simulink model "SD2231_Lab1_2022"  (R2020b)
settings: Solver=VariableStepAuto  StartTime=0.0  StopTime=inf  RelTol=1e-3
values from neighbouring files (symbols this model uses):
  delay = 250    [initial.m]
  K_awup = Ki_br_r/Kp_br_r    (= 10.4166666667)    [initial.m]
  K_brake = K_brake(3)    [initial.m]
  K_em = K_em(3)    [initial.m]
  Kd_br_f = 0*0.6*T_new_rl_b    (= 0)    [initial.m]
  Kd_br_r = 0.6*T_new_rl_b    (= 0.1722)    [initial.m]
  Kd_tr = 0.6*T_new    (= 0.0093)    [initial.m]
  Ki_br_f = 0.5*0.6*T_new_rl_b/L_new_rl_b^2    (= 37.3697916667)    [initial.m]
  Ki_br_r = 0.6*T_new_rl_b/L_new_rl_b^2    (= 74.7395833333)    [initial.m]
  Ki_tr = 0.6*T_new/L_new^2    (= 4.12188365651)    [initial.m]
  Kp_br_f = 1.2*T_new_rl_b/L_new_rl_b    (= 7.175)    [initial.m]
  Kp_br_r = 1.2*T_new_rl_b/L_new_rl_b    (= 7.175)    [initial.m]
  Kp_tr = 2.2*1.2*T_new/L_new    (= 0.861473684211)    [initial.m]
  N = 100    [initial.m]
  ref_br_f = 0.15    [initial.m]
  ref_br_r = 0.17-0.1    (= 0.07)    [initial.m]
  ref_tr = 0.06    [initial.m]
  step_time = 2    [initial.m]
  threshold_br_f = ref_br_f-0.05    (= 0.1)    [initial.m]
  threshold_br_r = ref_br_r-0.05    (= 0.02)    [initial.m]
  threshold_tc = ref_tr-0.02    (= 0.04)    [initial.m]
  vx_threshold = 1    [initial.m]
undefined symbols (not defined in the file or in its folder): DiscIntNeverNeededParam, Veh
libraries: CarMaker4SL x38, simulink x2, autolibmappedmotor x2
(part 4 of 4)

== system SD2231_Lab1_2022/CarMaker/IPG Vehicle/PowerTrain/User RearDriven PowerTrain1/RR Motor ==
  Gas : Inport
  "Motor speed " : Inport  Port=2
  Mapped Motor : autolibmappedmotor/Mapped Motor  port_config=Speed  param_by=Tabulated torque-speed envelope  w_t=[ 0 500 5000 10000 16000]  T_t=[440 440 350 300 280]  torque_max=.1  power_max=30  Tc=0.02  param_loss=Single efficiency measurement  eff=100  w_eff=375  T_eff=440  Piron=0  Pbase=0  w_eff_bp=[-8000 -4000 0 4000 8000]  T_eff_bp=[0 0.03 0.06 0.09]  Temp_eff_bp=[233.15 293.15 373.15]  losses_table=[1.49 1.67 2.21 3.10; 0.42 0.69 1.14 2.03; 0.06 0.24 0.78 1.68; 0.42 0.69 1.14 2.03; 1.49 1.67 2.21 3.10]  losses_table_3d=cat(3,1.05*[1.49 1.67 2.21 3.10; 0.42 0.69 1.14 2.03; 0.06 0.24 0.78 1.68; 0.42 0.69 1.14 2.03; 1.49 1.67 2.21 3.10],[1.49 1.67 2.21 3.10; 0.42 0.69 1.14 2.03; 0.06 0.24 0.78 1.68; 0.42 0.69 1.14 2.03; 1.49 1.67 2.21 3.10],1.03*[1.49 1.67 2.21 3.10; 0.42 0.69 1.14 2.03; 0.06 0.24 0.78 1.68; 0.42 0.69 1.14 2.03; 1.49 1.67 2.21 3.10])  efficiency_table=[95 95 95 95; 95 95 95 95; 95 95 95 95; 95 95 95 95; 95 95 95 95]  efficiency_table_3d=cat(3,90*ones(5,4),95*ones(5,4),92*ones(5,4))  J=0.002  b=1e-5  omega_o=0  T_t_extended=[280 300 350 440 440 440 350 300 280]  w_t_extended=[-16000 -10000 -5000 -500 0 500 5000 10000 16000]  KLossIron=0  KLossCopper=0  x_w_eff_vec=[-8000 -4000 0 4000 8000]  x_T_eff_vec=[-0.09 -0.06 -0.03 0 0.03 0.06 0.09]  x_tmp_eff_vec=[233.15 293.15 373.15]  x_losses_mat=[3.1 2.21 1.67 1.49 1.67 2.21 3.1;2.03 1.14 0.69 0.42 0.69 1.14 2.03;1.68 0.78 0.24 0.06 0.24 0.78 1.68;2.03 1.14 0.69 0.42 0.69 1.14 2.03;3.1 2.21 1.67 1.49 1.67 2.21 3.1]  x_losses_mat_3d=cat(3,[3.255 2.3205 1.7535 1.5645 1.7535 2.3205 3.255;2.1315 1.197 0.7245 0.441 0.7245 1.197 2.1315;1.764 0.819 0.252 0.063 0.252 0.819 1.764;2.1315 1.197 0.7245 0.441 0.7245 1.197 2.1315;3.255 2.3205 1.7535 1.5645 1.7535 2.3205 3.255],[3.1 2.21 1.67 1.49 1.67 2.21 3.1;2.03 1.14 0.69 0.42 0.69 1.14 2.03;1.68 0.78 0.24 0.06 0.24 0.78 1.68;2.03 1.14 0.69 0.42 0.69 1.14 2.03;3.1 2.21 1.67 1.49 1.67 2.21 3.1],[3.193 2.2763 1.7201 1.5347 1.7201 2.2763 3.193;2.0909 1.1742 0.7107 0.4326 0.7107 1.1742 2.0909;1.7304 0.8034 0.2472 0.0618 0.2472 0.8034 1.7304;2.0909 1.1742 0.7107 0.4326 0.7107 1.1742 2.0909;3.193 2.2763 1.7201 1.5347 1.7201 2.2763 3.193])  CalLossMapData={}  CalLossWithTempMapData={}  aMode=2  RefBlkName='autolibmappedmotor/Mapped Motor'
      settings: SourceProductBaseCode=PW
  "Max Torque from motor " : Constant  Value=K_em
  Product : Product  RndMeth=Zero
  Read CM Dict : CarMaker4SL/Read CM Dict  xname=PT.BattHV.Volt_oc  xsync=off  xstime=Continuous
  Scope : Scope
  Terminator : Terminator
  Terminator1 : Terminator
  Motor Trq : Outport  VectorParamsAs1DForOutWhenUnconnected=off
  wires:
  Mapped Motor/3 -> Motor Trq/1
  Read CM Dict/1 -> Mapped Motor/1
  Gas/1 -> Product/1
  Product/1 -> Mapped Motor/3
  "Max Torque from motor "/1 -> Product/2
  Mapped Motor/1 -> Terminator/1
  Mapped Motor/2 -> Terminator1/1
  "Motor speed "/1 -> Scope/1, Mapped Motor/2

== system SD2231_Lab1_2022/CarMaker/IPG Vehicle/PowerTrain/User RearDriven PowerTrain1/Subsystem ==
  LR motor Torque : Inport
  RR motor Torque : Inport  Port=2
  Gear ratio : Gain  Gain=9.73
  Gear ratio1 : Gain  Gain=9.73
  "LRTrq " : Outport  VectorParamsAs1DForOutWhenUnconnected=off
  RRTrq : Outport  Port=2  VectorParamsAs1DForOutWhenUnconnected=off
  wires:
  LR motor Torque/1 -> Gear ratio1/1
  RR motor Torque/1 -> Gear ratio/1
  Gear ratio/1 -> RRTrq/1
  Gear ratio1/1 -> "LRTrq "/1

== system SD2231_Lab1_2022/CarMaker/IPG Vehicle/PowerTrain/User RearDriven PowerTrain1/WheelInertia ==
  In1 : Inport
  Divide : Product  Inputs=*/
  Read CM Parameter : CarMaker4SL/Read CM Parameter  xfile=Vehicle  xkey=Wheel.fl.I  xnout=3  xdefaults=[]  xmuxed=off  xstime=Continuous
      settings: SourceProductName=CarMaker4SL
  Switch : Switch  Criteria=u2 ~= 0  ZeroCross=off
  Terminator : Terminator
  Terminator1 : Terminator
  Zero : Constant
  Out1 : Outport  VectorParamsAs1DForOutWhenUnconnected=off
  wires:
  Read CM Parameter/2 -> Switch/1, Switch/2
  Switch/1 -> Divide/2
  Zero/1 -> Switch/3
  In1/1 -> Divide/1
  Read CM Parameter/3 -> Terminator1/1
  Read CM Parameter/1 -> Terminator/1
  Divide/1 -> Out1/1

== system SD2231_Lab1_2022/CarMaker/IPG Vehicle/PowerTrain/User RearDriven PowerTrain1/WheelInertia1 ==
  In1 : Inport
  Divide : Product  Inputs=*/
  Read CM Parameter : CarMaker4SL/Read CM Parameter  xfile=Vehicle  xkey=Wheel.fr.I  xnout=3  xdefaults=[]  xmuxed=off  xstime=Continuous
      settings: SourceProductName=CarMaker4SL
  Switch : Switch  Criteria=u2 ~= 0  ZeroCross=off
  Terminator : Terminator
  Terminator1 : Terminator
  Zero : Constant
  Out1 : Outport  VectorParamsAs1DForOutWhenUnconnected=off
  wires:
  Divide/1 -> Out1/1
  Read CM Parameter/1 -> Terminator/1
  Read CM Parameter/3 -> Terminator1/1
  In1/1 -> Divide/1
  Read CM Parameter/2 -> Switch/2, Switch/1
  Zero/1 -> Switch/3
  Switch/1 -> Divide/2

== system SD2231_Lab1_2022/CarMaker/IPG Vehicle/PowerTrain/User RearDriven PowerTrain1/WheelInertia2 ==
  In1 : Inport
  Divide : Product  Inputs=*/
  Read CM Parameter : CarMaker4SL/Read CM Parameter  xfile=Vehicle  xkey=Wheel.rl.I  xnout=3  xdefaults=[]  xmuxed=off  xstime=Continuous
      settings: SourceProductName=CarMaker4SL
  Switch : Switch  Criteria=u2 ~= 0  ZeroCross=off
  Terminator : Terminator
  Terminator1 : Terminator
  Zero : Constant
  Out1 : Outport  VectorParamsAs1DForOutWhenUnconnected=off
  wires:
  Switch/1 -> Divide/2
  Zero/1 -> Switch/3
  Read CM Parameter/2 -> Switch/1, Switch/2
  In1/1 -> Divide/1
  Read CM Parameter/3 -> Terminator1/1
  Read CM Parameter/1 -> Terminator/1
  Divide/1 -> Out1/1

== system SD2231_Lab1_2022/CarMaker/IPG Vehicle/PowerTrain/User RearDriven PowerTrain1/WheelInertia3 ==
  In1 : Inport
  Divide : Product  Inputs=*/
  Read CM Parameter : CarMaker4SL/Read CM Parameter  xfile=Vehicle  xkey=Wheel.rr.I  xnout=3  xdefaults=[]  xmuxed=off  xstime=Continuous
      settings: SourceProductName=CarMaker4SL
  Switch : Switch  Criteria=u2 ~= 0  ZeroCross=off
  Terminator : Terminator
  Terminator1 : Terminator
  Zero : Constant
  Out1 : Outport  VectorParamsAs1DForOutWhenUnconnected=off
  wires:
  Divide/1 -> Out1/1
  Read CM Parameter/1 -> Terminator/1
  Read CM Parameter/3 -> Terminator1/1
  In1/1 -> Divide/1
  Read CM Parameter/2 -> Switch/2, Switch/1
  Zero/1 -> Switch/3
  Switch/1 -> Divide/2

== system SD2231_Lab1_2022/CarMaker/Your ABS Controller/Activation Logic Br FL/Subsystem/PID1 ==
  err : Inport
  Brake Pedal : Inport  Port=2
  slip : Inport  Port=3
  Add : Sum
  Add1 : Sum  Inputs=-+
  Add2 : Sum
  Brake Pedal1 : InportShadow  Port=2
  Constant : Constant  Value=0
  Constant1 : Constant  Value=0
  Constant2 : Constant  Value=threshold_br_f
  Integrator : Integrator
  Integrator1 : Integrator
  Kd : Gain  Gain=Kd_br_f
  Ki : Gain  Gain=Ki_br_f
  Ki1 : Gain  Gain=K_awup
  MATLAB Function : MATLAB Function  TreatAsAtomicUnit=on
  Manual Switch : ManualSwitch  CurrentSetting=0
  N : Gain  Gain=N
  PID FL : Scope  NumInputPorts=4
  Saturation : Saturate  UpperLimit=1  LowerLimit=0
  Scope1 : Scope  NumInputPorts=2
  Sum : Sum  Inputs=|+-
  Sum1 : Sum  Inputs=+|+|+
  Switch : Switch  Criteria=u2 > Threshold  Threshold=0.5
  kp : Gain  Gain=Kp_br_f
  AdjBrk : Outport
  wires:
  kp/1 -> PID FL/1, Sum1/1  "KP"
  Integrator1/1 -> Sum/2
  N/1 -> Integrator1/1, Sum1/3, PID FL/3  "KD"
  Sum/1 -> N/1
  Kd/1 -> Sum/1
  Integrator/1 -> PID FL/2, Sum1/2  "KI"
  err/1 -> Switch/1, PID FL/4, kp/1, Kd/1  "err"
  Sum1/1 -> Add/1, AdjBrk/1
  Brake Pedal/1 -> Add/2
  Add/1 -> Add1/1, Saturation/1
  Saturation/1 -> Add1/2
  Add1/1 -> Ki1/1
  Ki/1 -> Scope1/1, Add2/1
  Add2/1 -> Integrator/1
  Manual Switch/1 -> Add2/2
  Constant/1 -> Manual Switch/1
  Ki1/1 -> Scope1/2, Manual Switch/2
  Switch/1 -> Ki/1  "err_slip"
  Constant1/1 -> Switch/3
  MATLAB Function/1(res) -> Switch/2
  slip/1 -> MATLAB Function/2(slip)
  Brake Pedal1/1 -> MATLAB Function/3(Brk)
  Constant2/1 -> MATLAB Function/1(threshold_br_r)

== system SD2231_Lab1_2022/CarMaker/Your ABS Controller/Activation Logic Br FR/Subsystem/PID ==
  err : Inport
  res : Inport  Port=2
  Integrator : Integrator  ExternalReset=rising
  Integrator1 : Integrator
  Kd : Gain  Gain=Kd_br_f
  Ki : Gain  Gain=Ki_br_f
  N : Gain  Gain=N
  Sum : Sum  Inputs=|+-
  Sum1 : Sum  Inputs=+|+|+
  kp : Gain  Gain=Kp_br_f
  Out1 : Outport
  wires:
  err/1 -> Kd/1, Ki/1, kp/1
  Ki/1 -> Integrator/1
  Kd/1 -> Sum/1
  Sum/1 -> N/1
  N/1 -> Sum1/3, Integrator1/1
  Integrator1/1 -> Sum/2
  Integrator/1 -> Sum1/2
  kp/1 -> Sum1/1
  Sum1/1 -> Out1/1
  res/1 -> Integrator/2

== system SD2231_Lab1_2022/CarMaker/Your ABS Controller/Activation Logic Br FR/Subsystem1/PID1 ==
  err : Inport
  Brake Pedal : Inport  Port=2
  slip : Inport  Port=3
  Add : Sum
  Add1 : Sum  Inputs=-+
  Add2 : Sum
  Brake Pedal1 : InportShadow  Port=2
  Constant : Constant  Value=0
  Constant1 : Constant  Value=0
  Constant2 : Constant  Value=threshold_br_f
  Integrator : Integrator
  Integrator1 : Integrator
  Kd : Gain  Gain=Kd_br_f
  Ki : Gain  Gain=Ki_br_f
  Ki1 : Gain  Gain=K_awup
  MATLAB Function1 : MATLAB Function  TreatAsAtomicUnit=on
  Manual Switch : ManualSwitch  CurrentSetting=0
  N : Gain  Gain=N
  Saturation : Saturate  UpperLimit=1  LowerLimit=0
  Scope : Scope  NumInputPorts=4
  Scope1 : Scope  NumInputPorts=2
  Sum : Sum  Inputs=|+-
  Sum1 : Sum  Inputs=+|+|+
  Switch : Switch  Criteria=u2 > Threshold  Threshold=0.5
  kp : Gain  Gain=Kp_br_f
  AdjBrk : Outport
  wires:
  kp/1 -> Scope/1, Sum1/1  "KP"
  Integrator1/1 -> Sum/2
  N/1 -> Integrator1/1, Sum1/3, Scope/3  "KD"
  Sum/1 -> N/1
  Kd/1 -> Sum/1
  Integrator/1 -> Scope/2, Sum1/2  "KI"
  Sum1/1 -> Add/1, AdjBrk/1
  Brake Pedal/1 -> Add/2
  Add/1 -> Add1/1, Saturation/1
  Saturation/1 -> Add1/2
  Add1/1 -> Ki1/1
  Ki/1 -> Scope1/1, Add2/1
  Add2/1 -> Integrator/1
  Manual Switch/1 -> Add2/2
  Constant/1 -> Manual Switch/1
  Ki1/1 -> Scope1/2, Manual Switch/2
  Constant1/1 -> Switch/3
  err/1 -> Switch/1, Scope/4, kp/1, Kd/1  "err_slip"
  Switch/1 -> Ki/1  "err_slip"
  slip/1 -> MATLAB Function1/2(slip)
  Brake Pedal1/1 -> MATLAB Function1/3(Brk)
  MATLAB Function1/1(res) -> Switch/2
  Constant2/1 -> MATLAB Function1/1(threshold_br_r)

== system SD2231_Lab1_2022/CarMaker/Your ABS Controller/Activation Logic Br RL/Subsystem/PID1 ==
  err : Inport
  slip : Inport  Port=2
  Brake Pedal : Inport  Port=3
  Add : Sum
  Add1 : Sum  Inputs=-+
  Add2 : Sum
  Brake Pedal1 : InportShadow  Port=3
  Constant : Constant  Value=0
  Constant1 : Constant  Value=0
  Constant2 : Constant  Value=threshold_br_r
  Integrator : Integrator
  Integrator1 : Integrator
  Kd : Gain  Gain=Kd_br_r
  Ki : Gain  Gain=Ki_br_r
  Ki1 : Gain  Gain=K_awup
  MATLAB Function : MATLAB Function  TreatAsAtomicUnit=on
  Manual Switch : ManualSwitch  CurrentSetting=0
  N : Gain  Gain=N
  PID FL : Scope  NumInputPorts=4
  Saturation : Saturate  UpperLimit=1  LowerLimit=0
  Scope1 : Scope  NumInputPorts=2
  Sum : Sum  Inputs=|+-
  Sum1 : Sum  Inputs=+|+|+
  Switch : Switch  Criteria=u2 > Threshold  Threshold=0.5
  kp : Gain  Gain=Kp_br_r
  AdjBrk : Outport
  wires:
  kp/1 -> PID FL/1, Sum1/1  "KP"
  Integrator1/1 -> Sum/2
  N/1 -> Integrator1/1, Sum1/3, PID FL/3  "KD"
  Sum/1 -> N/1
  Kd/1 -> Sum/1
  Integrator/1 -> PID FL/2, Sum1/2  "KI"
  err/1 -> Switch/1, PID FL/4, kp/1, Kd/1  "err"
  Sum1/1 -> Add/1, AdjBrk/1
  Brake Pedal/1 -> Add/2
  Add/1 -> Add1/1, Saturation/1
  Saturation/1 -> Add1/2
  Add1/1 -> Ki1/1
  Ki/1 -> Scope1/1, Add2/1
  Add2/1 -> Integrator/1
  Manual Switch/1 -> Add2/2
  Constant/1 -> Manual Switch/1
  Ki1/1 -> Scope1/2, Manual Switch/2
  Switch/1 -> Ki/1  "err_slip"
  Constant1/1 -> Switch/3
  Brake Pedal1/1 -> MATLAB Function/3(Brk)
  MATLAB Function/1(res) -> Switch/2
  slip/1 -> MATLAB Function/2(slip)
  Constant2/1 -> MATLAB Function/1(threshold_br_r)  "threshold_br_r"

== system SD2231_Lab1_2022/CarMaker/Your ABS Controller/Activation Logic Br RL old/Subsystem/PID ==
  err : Inport
  res : Inport  Port=2
  Integrator : Integrator  ExternalReset=rising
  Integrator1 : Integrator
  Kd : Gain  Gain=Kd_br_r
  Ki : Gain  Gain=Ki_br_r
  N : Gain  Gain=N
  Sum : Sum  Inputs=|+-
  Sum1 : Sum  Inputs=+|+|+
  kp : Gain  Gain=Kp_br_r
  Out1 : Outport
  wires:
  err/1 -> Kd/1, Ki/1, kp/1
  Ki/1 -> Integrator/1
  Kd/1 -> Sum/1
  Sum/1 -> N/1
  N/1 -> Sum1/3, Integrator1/1
  Integrator1/1 -> Sum/2
  Integrator/1 -> Sum1/2
  kp/1 -> Sum1/1
  Sum1/1 -> Out1/1
  res/1 -> Integrator/2

== system SD2231_Lab1_2022/CarMaker/Your ABS Controller/Activation Logic Br RL old 2/Controller/PID ==
  err : Inport
  Brake Pedal : Inport  Port=2
  Add : Sum
  Add1 : Sum  Inputs=-+
  Add2 : Sum
  Brake Pedal1 : InportShadow  Port=2
  Constant : Constant  Value=0
  Constant1 : Constant  Value=0
  Integrator : Integrator
  Integrator1 : Integrator
  Kd : Gain  Gain=Kd_br_r
  Ki : Gain  Gain=Ki_br_r
  Ki1 : Gain  Gain=K_awup
  MATLAB Function : MATLAB Function  TreatAsAtomicUnit=on
  Manual Switch : ManualSwitch
  N : Gain  Gain=N
  PID RL : Scope  NumInputPorts=4
  Saturation : Saturate  UpperLimit=1  LowerLimit=0
  Scope : Scope
  Sum : Sum  Inputs=|+-
  Sum1 : Sum  Inputs=+|+|+
  Switch : Switch  Criteria=u2 > Threshold  Threshold=0.5
  kp : Gain  Gain=Kp_br_r
  AdjBrk : Outport
  wires:
  Constant/1 -> Manual Switch/1
  Manual Switch/1 -> Add2/2
  Ki1/1 -> Manual Switch/2
  Add2/1 -> Integrator/1
  Ki/1 -> Add2/1
  Add1/1 -> Ki1/1
  Saturation/1 -> Add1/2
  Add/1 -> Saturation/1, Add1/1
  Brake Pedal/1 -> Add/2
  Sum1/1 -> AdjBrk/1, Add/1
  Integrator/1 -> Sum1/2, PID RL/2  "KI"
  Kd/1 -> Sum/1
  Sum/1 -> N/1
  N/1 -> PID RL/3, Sum1/3, Integrator1/1  "KD"
  Integrator1/1 -> Sum/2
  kp/1 -> Sum1/1, PID RL/1  "KP"
  err/1 -> Kd/1, kp/1, PID RL/4, Switch/1  "err_slip"
  MATLAB Function/1(res) -> Switch/2
  Constant1/1 -> Switch/3
  Brake Pedal1/1 -> MATLAB Function/1(Brk)
  Switch/1 -> Scope/1, Ki/1

== system SD2231_Lab1_2022/CarMaker/Your ABS Controller/Activation Logic Br RR/Subsystem/PID1 ==
  err : Inport
  slip : Inport  Port=2
  Brake Pedal : Inport  Port=3
  Add : Sum
  Add1 : Sum  Inputs=-+
  Add2 : Sum
  Brake Pedal1 : InportShadow  Port=3
  Constant : Constant  Value=0
  Constant1 : Constant  Value=0
  Constant2 : Constant  Value=threshold_br_r
  Integrator : Integrator
  Integrator1 : Integrator
  Kd : Gain  Gain=Kd_br_r
  Ki : Gain  Gain=Ki_br_r
  Ki1 : Gain  Gain=K_awup
  MATLAB Function : MATLAB Function  TreatAsAtomicUnit=on
  Manual Switch : ManualSwitch  CurrentSetting=0
  N : Gain  Gain=N
  PID Br RR : Scope  NumInputPorts=4
  Saturation : Saturate  UpperLimit=1  LowerLimit=0
  Scope1 : Scope  NumInputPorts=2
  Sum : Sum  Inputs=|+-
  Sum1 : Sum  Inputs=+|+|+
  Switch : Switch  Criteria=u2 > Threshold  Threshold=0.5
  kp : Gain  Gain=Kp_br_r
  AdjBrk : Outport
  wires:
  MATLAB Function/1(res) -> Switch/2
  Brake Pedal1/1 -> MATLAB Function/3(Brk)
  Constant1/1 -> Switch/3
  Switch/1 -> Ki/1  "err_slip"
  Ki1/1 -> Manual Switch/2, Scope1/2
  Constant/1 -> Manual Switch/1
  Manual Switch/1 -> Add2/2
  Add2/1 -> Integrator/1
  Ki/1 -> Add2/1, Scope1/1
  Add1/1 -> Ki1/1
  Saturation/1 -> Add1/2
  Add/1 -> Saturation/1, Add1/1
  Brake Pedal/1 -> Add/2
  Sum1/1 -> AdjBrk/1, Add/1
  err/1 -> Kd/1, kp/1, PID Br RR/4, Switch/1  "err"
  Integrator/1 -> Sum1/2, PID Br RR/2  "KI"
  Kd/1 -> Sum/1
  Sum/1 -> N/1
  N/1 -> PID Br RR/3, Sum1/3, Integrator1/1  "KD"
  Integrator1/1 -> Sum/2
  kp/1 -> Sum1/1, PID Br RR/1  "KP"
  slip/1 -> MATLAB Function/2(slip)
  Constant2/1 -> MATLAB Function/1(threshold_br_r)

== system SD2231_Lab1_2022/CarMaker/Your ABS Controller/Activation Logic Br RR old 2/Controller/PID ==
  note: D
  err : Inport
  Brake Pedal : Inport  Port=2
  Add : Sum
  Add1 : Sum  Inputs=-+
  Add2 : Sum
  Add3 : Sum  Inputs=+-
  Brake Pedal1 : InportShadow  Port=2
  Constant : Constant  Value=0
  Constant1 : Constant  Value=0
  Integrator : Integrator
  Integrator1 : Integrator
  Kd : Gain  Gain=Kd_br_r
  Ki : Gain  Gain=Ki_br_r
  Ki1 : Gain  Gain=K_awup
  MATLAB Function : MATLAB Function  TreatAsAtomicUnit=on
  Manual Switch : ManualSwitch  CurrentSetting=0
  N : Gain  Gain=N
  Saturation : Saturate  UpperLimit=1  LowerLimit=0
  Scope : Scope  NumInputPorts=5
  Scope1 : Scope  NumInputPorts=2
  Sum : Sum  Inputs=|+-
  Sum1 : Sum  Inputs=+|+|+
  Switch : Switch  Criteria=u2 > Threshold  Threshold=0.5
  kp : Gain  Gain=Kp_br_r
  AdjBrk : Outport
  wires:
  kp/1 -> Scope/1, Sum1/1  "KP"
  Integrator1/1 -> Sum/2
  N/1 -> Sum1/3, Scope/4, Integrator1/1  "KD"
  Sum/1 -> N/1
  Kd/1 -> Sum/1
  Integrator/1 -> Scope/3, Sum1/2  "KI"
  err/1 -> Switch/1, Kd/1, kp/1, Scope/5  "err"
  Sum1/1 -> Scope/2, AdjBrk/1, Add/1
  Brake Pedal/1 -> Add3/2, Add/2
  Add/1 -> Saturation/1, Add1/1
  Saturation/1 -> Add1/2
  Add1/1 -> Ki1/1
  Ki/1 -> Scope1/1, Add2/1
  Add2/1 -> Integrator/1
  Manual Switch/1 -> Add2/2
  Constant/1 -> Manual Switch/1
  Ki1/1 -> Add3/1
  Add3/1 -> Scope1/2, Manual Switch/2
  MATLAB Function/1(res) -> Switch/2
  Constant1/1 -> Switch/3
  Switch/1 -> Ki/1
  Brake Pedal1/1 -> MATLAB Function/1(Brk)

== system SD2231_Lab1_2022/CarMaker/Your ABS Controller/Activation Logic1/Subsystem/PID ==
  err : Inport
  Integrator : Integrator
  Integrator1 : Integrator
  Kd : Gain  Gain=Kd_br_f
  Ki : Gain  Gain=Ki_br_f
  N : Gain  Gain=N
  Sum : Sum  Inputs=|+-
  Sum1 : Sum  Inputs=+|+|+
  kp : Gain  Gain=Kp_br_f
  Out1 : Outport
  wires:
  err/1 -> Kd/1, Ki/1, kp/1
  Ki/1 -> Integrator/1
  Kd/1 -> Sum/1
  Sum/1 -> N/1
  N/1 -> Sum1/3, Integrator1/1
  Integrator1/1 -> Sum/2
  Integrator/1 -> Sum1/2
  kp/1 -> Sum1/1
  Sum1/1 -> Out1/1

== system SD2231_Lab1_2022/CarMaker/Your ABS Controller/Activation Logic1/Subsystem1/PID ==
  err : Inport
  y : Inport  Port=2
  Integrator : Integrator  ExternalReset=falling
  Integrator1 : Integrator
  Kd : Gain  Gain=Kd_br_f
  Ki : Gain  Gain=Ki_br_f
  N : Gain  Gain=N
  Sum : Sum  Inputs=|+-
  Sum1 : Sum  Inputs=+|+|+
  kp : Gain  Gain=Kp_br_f
  Out1 : Outport
  wires:
  err/1 -> Ki/1, kp/1, Kd/1
  Ki/1 -> Integrator/1
  Kd/1 -> Sum/1
  Sum/1 -> N/1
  N/1 -> Sum1/3, Integrator1/1
  Integrator1/1 -> Sum/2
  Integrator/1 -> Sum1/2
  kp/1 -> Sum1/1
  Sum1/1 -> Out1/1
  y/1 -> Integrator/2

== system SD2231_Lab1_2022/CarMaker/Your Traction Controller/Activation Logic RL tr1/Subsystem/PID ==
  err : Inport
  Integrator : Integrator
  Integrator1 : Integrator
  Kd : Gain  Gain=Kd_br_f
  Ki : Gain  Gain=Ki_br_f
  N : Gain  Gain=N
  Sum : Sum  Inputs=|+-
  Sum1 : Sum  Inputs=+|+|+
  kp : Gain  Gain=Kp_br_f
  Out1 : Outport
  wires:
  Sum1/1 -> Out1/1
  kp/1 -> Sum1/1
  Integrator/1 -> Sum1/2
  Integrator1/1 -> Sum/2
  N/1 -> Integrator1/1, Sum1/3
  Sum/1 -> N/1
  Kd/1 -> Sum/1
  Ki/1 -> Integrator/1
  err/1 -> kp/1, Ki/1, Kd/1

== system SD2231_Lab1_2022/CarMaker/Your Traction Controller/Activation Logic RL tr1/Subsystem1/PID ==
  err : Inport
  Integrator : Integrator
  Integrator1 : Integrator
  Kd : Gain  Gain=Kd_tr
  Ki : Gain  Gain=Ki_tr
  N : Gain  Gain=N
  Sum : Sum  Inputs=|+-
  Sum1 : Sum  Inputs=+|+|+
  kp : Gain  Gain=Kp_tr
  Out1 : Outport
  wires:
  Sum1/1 -> Out1/1
  kp/1 -> Sum1/1
  Integrator/1 -> Sum1/2
  Integrator1/1 -> Sum/2
  N/1 -> Integrator1/1, Sum1/3
  Sum/1 -> N/1
  Kd/1 -> Sum/1
  Ki/1 -> Integrator/1
  err/1 -> Kd/1, kp/1, Ki/1

== system SD2231_Lab1_2022/CarMaker/Your Traction Controller/Activation Logic RL tr2/Subsystem/PID ==
  err : Inport
  Integrator : Integrator
  Integrator1 : Integrator
  Kd : Gain  Gain=Kd_br_f
  Ki : Gain  Gain=Ki_br_f
  N : Gain  Gain=N
  Sum : Sum  Inputs=|+-
  Sum1 : Sum  Inputs=+|+|+
  kp : Gain  Gain=Kp_br_f
  Out1 : Outport
  wires:
  Sum1/1 -> Out1/1
  kp/1 -> Sum1/1
  Integrator/1 -> Sum1/2
  Integrator1/1 -> Sum/2
  N/1 -> Integrator1/1, Sum1/3
  Sum/1 -> N/1
  Kd/1 -> Sum/1
  Ki/1 -> Integrator/1
  err/1 -> kp/1, Ki/1, Kd/1

== system SD2231_Lab1_2022/CarMaker/Your Traction Controller/Activation Logic RL tr2/Subsystem2/PID ==
  err : Inport
  Integrator : Integrator
  Integrator1 : Integrator
  Kd : Gain  Gain=Kd_tr
  Ki : Gain  Gain=Ki_tr
  N : Gain  Gain=N
  Sum : Sum  Inputs=|+-
  Sum1 : Sum  Inputs=+|+|+
  kp : Gain  Gain=Kp_tr
  Out1 : Outport
  wires:
  err/1 -> Ki/1, kp/1, Kd/1
  Ki/1 -> Integrator/1
  Kd/1 -> Sum/1
  Sum/1 -> N/1
  N/1 -> Sum1/3, Integrator1/1
  Integrator1/1 -> Sum/2
  Integrator/1 -> Sum1/2
  kp/1 -> Sum1/1
  Sum1/1 -> Out1/1

== system SD2231_Lab1_2022/CarMaker/Your Traction Controller/Activation Logic Tr RL/Subsystem/PID ==
  err : Inport
  slip : Inport  Port=2
  <Throttle> : Inport  Port=3
  Constant : Constant  Value=threshold_tc
  Constant1 : Constant  Value=0
  Integrator : Integrator
  Integrator1 : Integrator
  Kd : Gain  Gain=Kd_tr
  Ki : Gain  Gain=Ki_tr
  MATLAB Function1 : MATLAB Function  TreatAsAtomicUnit=on
  N : Gain  Gain=N
  Sum : Sum  Inputs=|+-
  Sum1 : Sum  Inputs=+|+|+
  Switch : Switch  Criteria=u2 > Threshold  Threshold=0.5
  kp : Gain  Gain=Kp_tr
  AdjThr : Outport
  wires:
  Sum1/1 -> AdjThr/1
  kp/1 -> Sum1/1
  Integrator/1 -> Sum1/2
  Integrator1/1 -> Sum/2
  N/1 -> Integrator1/1, Sum1/3
  Sum/1 -> N/1
  Kd/1 -> Sum/1
  Ki/1 -> Integrator/1
  Constant/1 -> MATLAB Function1/2(threshold)
  <Throttle>/1 -> MATLAB Function1/1(Thr)
  slip/1 -> MATLAB Function1/3(slip)
  MATLAB Function1/1(res) -> Switch/2
  err/1 -> Kd/1, kp/1, Switch/1
  Switch/1 -> Ki/1
  Constant1/1 -> Switch/3

== system SD2231_Lab1_2022/CarMaker/Your Traction Controller/Activation Logic Tr RR/Controller/PID ==
  err : Inport
  res : Inport  Port=2
  Integrator : Integrator  ExternalReset=rising
  Integrator1 : Integrator  ExternalReset=rising
  Kd : Gain  Gain=Kd_tr
  Ki : Gain  Gain=Ki_tr
  N : Gain  Gain=N
  Sum : Sum  Inputs=|+-
  Sum1 : Sum  Inputs=+|+|+
  kp : Gain  Gain=Kp_tr
  Out1 : Outport
  wires:
  Sum1/1 -> Out1/1
  kp/1 -> Sum1/1
  Integrator/1 -> Sum1/2
  Integrator1/1 -> Sum/2
  N/1 -> Integrator1/1, Sum1/3
  Sum/1 -> N/1
  Kd/1 -> Sum/1
  Ki/1 -> Integrator/1
  err/1 -> kp/1, Ki/1, Kd/1
  res/1 -> Integrator1/2, Integrator/2

== system SD2231_Lab1_2022/CarMaker/Your Traction Controller/Activation Logic Tr RR/Subsystem/PID ==
  err : Inport
  slip : Inport  Port=2
  <Throttle> : Inport  Port=3
  Constant : Constant  Value=threshold_tc
  Constant1 : Constant  Value=0
  Integrator : Integrator
  Integrator1 : Integrator
  Kd : Gain  Gain=Kd_tr
  Ki : Gain  Gain=Ki_tr
  MATLAB Function1 : MATLAB Function  TreatAsAtomicUnit=on
  N : Gain  Gain=N
  PID tr RR : Scope  NumInputPorts=3
  Sum : Sum  Inputs=|+-
  Sum1 : Sum  Inputs=+|+|+
  Switch : Switch  Criteria=u2 > Threshold  Threshold=0.5
  kp : Gain  Gain=Kp_tr
  AdjThr : Outport
  wires:
  Sum1/1 -> AdjThr/1
  kp/1 -> PID tr RR/1, Sum1/1  "Kp"
  Integrator/1 -> PID tr RR/2, Sum1/2  "Ki"
  Integrator1/1 -> Sum/2
  N/1 -> Integrator1/1, PID tr RR/3, Sum1/3  "Kd"
  Sum/1 -> N/1
  Kd/1 -> Sum/1
  Ki/1 -> Integrator/1
  Constant/1 -> MATLAB Function1/2(threshold)
  <Throttle>/1 -> MATLAB Function1/1(Thr)
  slip/1 -> MATLAB Function1/3(slip)
  MATLAB Function1/1(res) -> Switch/2
  err/1 -> Kd/1, kp/1, Switch/1
  Switch/1 -> Ki/1
  Constant1/1 -> Switch/3

== system SD2231_Lab1_2022/CarMaker/Your Traction Controller/Activation Logic1/Subsystem/PID ==
  err : Inport
  Integrator : Integrator
  Integrator1 : Integrator
  Kd : Gain  Gain=Kd_tr
  Ki : Gain  Gain=Ki_tr
  N : Gain  Gain=N
  Sum : Sum  Inputs=|+-
  Sum1 : Sum  Inputs=+|+|+
  kp : Gain  Gain=Kp_tr
  Out1 : Outport
  wires:
  err/1 -> Kd/1, Ki/1, kp/1
  Ki/1 -> Integrator/1
  Kd/1 -> Sum/1
  Sum/1 -> N/1
  N/1 -> Sum1/3, Integrator1/1
  Integrator1/1 -> Sum/2
  Integrator/1 -> Sum1/2
  kp/1 -> Sum1/1
  Sum1/1 -> Out1/1

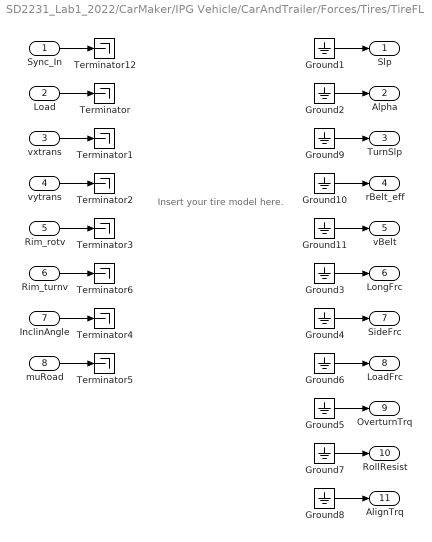
== system SD2231_Lab1_2022/CarMaker/IPG Vehicle/CarAndTrailer/Forces/Tires/TireFL ==
  note: Insert your tire model here.
  Sync_In : Inport
  Load : Inport  Port=2
  vxtrans : Inport  Port=3
  vytrans : Inport  Port=4
  Rim_rotv : Inport  Port=5
  Rim_turnv : Inport  Port=6
  InclinAngle : Inport  Port=7
  muRoad : Inport  Port=8
  Ground{1..11} (11 alike) : Ground
  Terminator{,1..6,12} (8 alike) : Terminator
  Slp : Outport
  Alpha : Outport  Port=2
  TurnSlp : Outport  Port=3
  rBelt_eff : Outport  Port=4
  vBelt : Outport  Port=5
  LongFrc : Outport  Port=6
  SideFrc : Outport  Port=7
  LoadFrc : Outport  Port=8
  OverturnTrq : Outport  Port=9
  RollResist : Outport  Port=10
  AlignTrq : Outport  Port=11
  wires:
  Ground11/1 -> vBelt/1
  Ground10/1 -> rBelt_eff/1
  Ground9/1 -> TurnSlp/1
  Rim_turnv/1 -> Terminator6/1
  Sync_In/1 -> Terminator12/1
  Ground2/1 -> Alpha/1
  Ground3/1 -> LongFrc/1
  Ground4/1 -> SideFrc/1
  Ground5/1 -> OverturnTrq/1
  vxtrans/1 -> Terminator1/1
  vytrans/1 -> Terminator2/1
  Rim_rotv/1 -> Terminator3/1
  InclinAngle/1 -> Terminator4/1
  muRoad/1 -> Terminator5/1
  Load/1 -> Terminator/1
  Ground1/1 -> Slp/1
  Ground6/1 -> LoadFrc/1
  Ground7/1 -> RollResist/1
  Ground8/1 -> AlignTrq/1

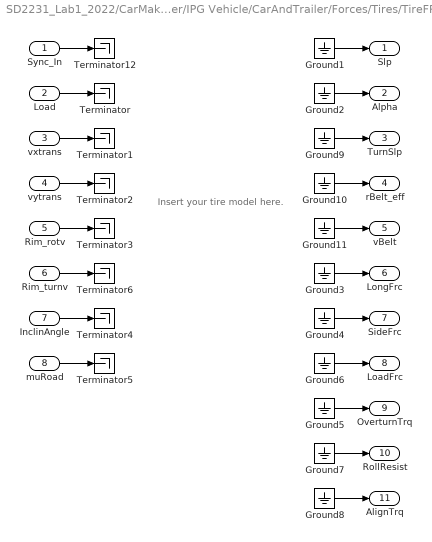
== system SD2231_Lab1_2022/CarMaker/IPG Vehicle/CarAndTrailer/Forces/Tires/TireFR ==
  note: Insert your tire model here.
  Sync_In : Inport
  Load : Inport  Port=2
  vxtrans : Inport  Port=3
  vytrans : Inport  Port=4
  Rim_rotv : Inport  Port=5
  Rim_turnv : Inport  Port=6
  InclinAngle : Inport  Port=7
  muRoad : Inport  Port=8
  Ground{1..11} (11 alike) : Ground
  Terminator{,1..6,12} (8 alike) : Terminator
  Slp : Outport
  Alpha : Outport  Port=2
  TurnSlp : Outport  Port=3
  rBelt_eff : Outport  Port=4
  vBelt : Outport  Port=5
  LongFrc : Outport  Port=6
  SideFrc : Outport  Port=7
  LoadFrc : Outport  Port=8
  OverturnTrq : Outport  Port=9
  RollResist : Outport  Port=10
  AlignTrq : Outport  Port=11
  wires:
  Ground11/1 -> vBelt/1
  Ground10/1 -> rBelt_eff/1
  Ground9/1 -> TurnSlp/1
  Rim_turnv/1 -> Terminator6/1
  Sync_In/1 -> Terminator12/1
  Ground2/1 -> Alpha/1
  Ground3/1 -> LongFrc/1
  Ground4/1 -> SideFrc/1
  Ground5/1 -> OverturnTrq/1
  vxtrans/1 -> Terminator1/1
  vytrans/1 -> Terminator2/1
  Rim_rotv/1 -> Terminator3/1
  InclinAngle/1 -> Terminator4/1
  muRoad/1 -> Terminator5/1
  Load/1 -> Terminator/1
  Ground1/1 -> Slp/1
  Ground6/1 -> LoadFrc/1
  Ground7/1 -> RollResist/1
  Ground8/1 -> AlignTrq/1

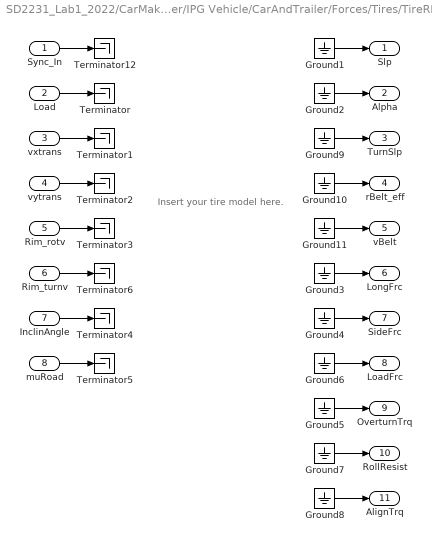
== system SD2231_Lab1_2022/CarMaker/IPG Vehicle/CarAndTrailer/Forces/Tires/TireRL ==
  note: Insert your tire model here.
  Sync_In : Inport
  Load : Inport  Port=2
  vxtrans : Inport  Port=3
  vytrans : Inport  Port=4
  Rim_rotv : Inport  Port=5
  Rim_turnv : Inport  Port=6
  InclinAngle : Inport  Port=7
  muRoad : Inport  Port=8
  Ground{1..11} (11 alike) : Ground
  Terminator{,1..6,12} (8 alike) : Terminator
  Slp : Outport
  Alpha : Outport  Port=2
  TurnSlp : Outport  Port=3
  rBelt_eff : Outport  Port=4
  vBelt : Outport  Port=5
  LongFrc : Outport  Port=6
  SideFrc : Outport  Port=7
  LoadFrc : Outport  Port=8
  OverturnTrq : Outport  Port=9
  RollResist : Outport  Port=10
  AlignTrq : Outport  Port=11
  wires:
  Ground11/1 -> vBelt/1
  Ground10/1 -> rBelt_eff/1
  Ground9/1 -> TurnSlp/1
  Rim_turnv/1 -> Terminator6/1
  Sync_In/1 -> Terminator12/1
  Ground2/1 -> Alpha/1
  Ground3/1 -> LongFrc/1
  Ground4/1 -> SideFrc/1
  Ground5/1 -> OverturnTrq/1
  vxtrans/1 -> Terminator1/1
  vytrans/1 -> Terminator2/1
  Rim_rotv/1 -> Terminator3/1
  InclinAngle/1 -> Terminator4/1
  muRoad/1 -> Terminator5/1
  Load/1 -> Terminator/1
  Ground1/1 -> Slp/1
  Ground6/1 -> LoadFrc/1
  Ground7/1 -> RollResist/1
  Ground8/1 -> AlignTrq/1

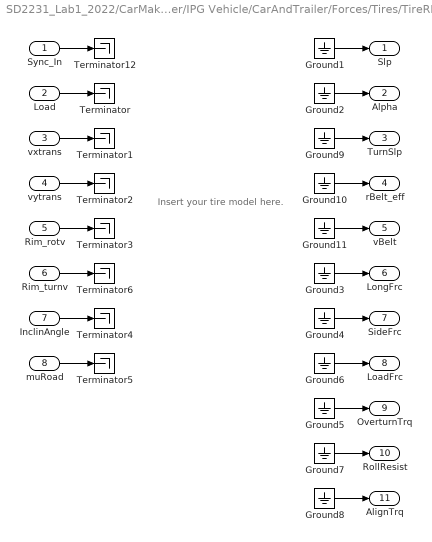
== system SD2231_Lab1_2022/CarMaker/IPG Vehicle/CarAndTrailer/Forces/Tires/TireRR ==
  note: Insert your tire model here.
  Sync_In : Inport
  Load : Inport  Port=2
  vxtrans : Inport  Port=3
  vytrans : Inport  Port=4
  Rim_rotv : Inport  Port=5
  Rim_turnv : Inport  Port=6
  InclinAngle : Inport  Port=7
  muRoad : Inport  Port=8
  Ground{1..11} (11 alike) : Ground
  Terminator{,1..6,12} (8 alike) : Terminator
  Slp : Outport
  Alpha : Outport  Port=2
  TurnSlp : Outport  Port=3
  rBelt_eff : Outport  Port=4
  vBelt : Outport  Port=5
  LongFrc : Outport  Port=6
  SideFrc : Outport  Port=7
  LoadFrc : Outport  Port=8
  OverturnTrq : Outport  Port=9
  RollResist : Outport  Port=10
  AlignTrq : Outport  Port=11
  wires:
  Ground11/1 -> vBelt/1
  Ground10/1 -> rBelt_eff/1
  Ground9/1 -> TurnSlp/1
  Rim_turnv/1 -> Terminator6/1
  Sync_In/1 -> Terminator12/1
  Ground2/1 -> Alpha/1
  Ground3/1 -> LongFrc/1
  Ground4/1 -> SideFrc/1
  Ground5/1 -> OverturnTrq/1
  vxtrans/1 -> Terminator1/1
  vytrans/1 -> Terminator2/1
  Rim_rotv/1 -> Terminator3/1
  InclinAngle/1 -> Terminator4/1
  muRoad/1 -> Terminator5/1
  Load/1 -> Terminator/1
  Ground1/1 -> Slp/1
  Ground6/1 -> LoadFrc/1
  Ground7/1 -> RollResist/1
  Ground8/1 -> AlignTrq/1

== matlab function SD2231_Lab1_2022/CarMaker/Your ABS Controller/Activation Logic Br FR/MATLAB Function ==
  data: vx input; ax input; Brk input; slip input; AdjBrk input; y output; threshold input; vx_threshold input
function y = fcn(vx, ax, Brk,slip,AdjBrk, threshold,vx_threshold)
if Brk > 0 && ax <0 && slip > threshold && vx > vx_threshold
    if AdjBrk > 0
        AdjBrk = 0;
    end
    y = AdjBrk+Brk;
else 
    y = Brk; %For later, try without this line
end

== matlab function SD2231_Lab1_2022/CarMaker/Your Traction Controller/Activation Logic1/MATLAB Function ==
  data: ax input; Thr input; slip input; AdjThr input; y output; threshold input
function y = fcn(ax, Thr,slip,AdjThr,threshold)
if Thr > 0 && ax >0 && slip > threshold 
    y = AdjThr;
else 
    y = Thr; %For later, try without this line
end

== matlab function SD2231_Lab1_2022/CarMaker/Your ABS Controller/Activation Logic Br FR/Subsystem/MATLAB Function ==
  data: Brk input; res output
function res = fcn(Brk)
if Brk >0
    res = 1;
else
    res = 0;
end
end

== matlab function SD2231_Lab1_2022/CarMaker/Your ABS Controller/Activation Logic Br RL old 2/Controller/PID/MATLAB Function ==
  data: Brk input; res output
function res = fcn(Brk)
if Brk >0
    res = 1;
else
    res = 0;
end
end

== matlab function SD2231_Lab1_2022/CarMaker/Your ABS Controller/Activation Logic Br RL old/Subsystem/MATLAB Function ==
  data: Brk input; res output
function res = fcn(Brk)
if Brk >0
    res = 1;
else
    res = 0;
end
end

== matlab function SD2231_Lab1_2022/CarMaker/Your ABS Controller/Activation Logic1/MATLAB Function ==
  data: ax input; vx input; Brk input; slip input; AdjBrk input; y output; threshold input
function y = fcn(ax, vx, Brk,slip,AdjBrk, threshold)
if Brk > 0 && ax <0 && slip > threshold && vx>0.5
    y = AdjBrk;
else 
    y = Brk; %For later, try without this line
end

== matlab function SD2231_Lab1_2022/CarMaker/Your ABS Controller/Activation Logic1/MATLAB Function1 ==
  data: s output; ax input; vx input; slip input; threshold input; Brk input; y output
function [s,y] = fcn(ax, vx,slip,threshold,Brk)
    s=slip;
if Brk > 0 && ax <0 && slip > threshold && vx > 0.5
    y = 1;
    
else 
    y = 0; 
end
% 1  = controller is ACTIVE
% 0 = controller is NOT ACTIVE

== matlab function SD2231_Lab1_2022/CarMaker/Your ABS Controller/Activation Logic Br RL old 2/MATLAB Function ==
  data: vx input; ax input; Brk input; slip input; AdjBrk input; y output; threshold input; vx_threshold input
function y = fcn(vx, ax, Brk,slip,AdjBrk, threshold,vx_threshold)
if Brk > 0 && ax <0 && slip > threshold && vx > vx_threshold
        if AdjBrk > 0
            AdjBrk = 0;
        end
    y = AdjBrk+Brk;
else 
    y = Brk; %For later, try without this line
end

== matlab function SD2231_Lab1_2022/CarMaker/Your Traction Controller/Activation Logic Tr RR/Subsystem/PID/MATLAB Function1 ==
  data: Thr input; res output; threshold input; slip input
function res = fcn(Thr,threshold,slip)
if Thr >0 && slip > threshold
    res = 1;
else
    res = 0;
end
end

== matlab function SD2231_Lab1_2022/CarMaker/Your ABS Controller/Activation Logic Br RL old/MATLAB Function ==
  data: vx input; ax input; Brk input; slip input; AdjBrk input; y output; threshold input; vx_threshold input
function y = fcn(vx, ax, Brk,slip,AdjBrk, threshold,vx_threshold)
if Brk > 0 && ax <0 && slip > threshold && vx > vx_threshold
    if AdjBrk > 0
        AdjBrk = 0;
    end
    y = AdjBrk+Brk;
else 
    y = Brk; %For later, try without this line
end

== matlab function SD2231_Lab1_2022/CarMaker/Your ABS Controller/Activation Logic Br RL/MATLAB Function ==
  data: vx input; ax input; Brk input; slip input; AdjBrk input; y output; threshold input; vx_threshold input
function y = fcn(vx, ax, Brk,slip,AdjBrk, threshold,vx_threshold)
if Brk > 0 && ax <0 && slip > threshold && vx > vx_threshold
    if AdjBrk > 0
        AdjBrk = 0;
    end
    y = AdjBrk+Brk;
else 
    y = Brk; %For later, try without this line
end

== matlab function SD2231_Lab1_2022/CarMaker/Your ABS Controller/Activation Logic Br RR old 2/Controller/PID/MATLAB Function ==
  data: Brk input; res output
function res = fcn(Brk)
if Brk >0
    res = 1;
else
    res = 0;
end
end

== matlab function SD2231_Lab1_2022/CarMaker/Your ABS Controller/Activation Logic Br RL/Subsystem/PID1/MATLAB Function ==
  data: threshold_br_r input; slip input; Brk input; res output
function res = fcn(threshold_br_r, slip, Brk)
if Brk >0 && slip > threshold_br_r
    res = 1;
else
    res = 0;
end
end

== matlab function SD2231_Lab1_2022/CarMaker/Your Traction Controller/Activation Logic RL tr1/MATLAB Function ==
  data: ax input; vx input; Brk input; slip input; AdjBrk input; y output; threshold input
function y = fcn(ax, vx, Brk,slip,AdjBrk, threshold)
if Brk > 0 && ax <0 && slip > threshold && vx>0.5
    y = AdjBrk;
else 
    y = Brk; %For later, try without this line
end

== matlab function SD2231_Lab1_2022/CarMaker/Your Traction Controller/Activation Logic RL tr1/MATLAB Function1 ==
  data: s output; ax input; vx input; slip input; threshold input; Thr input; y output
function [s,y] = fcn(ax, vx,slip,threshold,Thr)
    s=slip;
if Thr > 0 && ax >0 && slip > threshold && vx > 0.5
    y = 1;
    
else
    y = 0; 
end
% 1  = controller is ACTIVE
% 0 = controller is NOT ACTIVE

== matlab function SD2231_Lab1_2022/CarMaker/Your Traction Controller/Activation Logic RL tr2/MATLAB Function ==
  data: ax input; vx input; Brk input; slip input; AdjBrk input; y output; threshold input
function y = fcn(ax, vx, Brk,slip,AdjBrk, threshold)
if Brk > 0 && ax <0 && slip > threshold && vx>0.5
    y = AdjBrk;
else 
    y = Brk; %For later, try without this line
end

== matlab function SD2231_Lab1_2022/CarMaker/Your Traction Controller/Activation Logic RL tr2/MATLAB Function1 ==
  data: ax input; vx input; slip input; threshold input; Thr input; y output
function y  = fcn(ax, vx,slip,threshold,Thr)
    if Thr >0 && ax > 0 && slip > threshold
        y = 1
    
    


end
% 1  = controller is ACTIVE
% 0 = controller is NOT ACTIVE

== matlab function SD2231_Lab1_2022/CarMaker/Your ABS Controller/Activation Logic Br RR/MATLAB Function ==
  data: vx input; ax input; Brk input; slip input; AdjBrk input; y output; threshold input; vx_threshold input
function y = fcn(vx, ax, Brk,slip,AdjBrk, threshold,vx_threshold)
if Brk > 0 && ax <0 && slip > threshold && vx > vx_threshold
    if AdjBrk > 0
        AdjBrk = 0;
    end
    y = AdjBrk+Brk;
else 
    y = Brk; %For later, try without this line
end

== matlab function SD2231_Lab1_2022/CarMaker/Your Traction Controller/Activation Logic Tr RL/MATLAB Function ==
  settings: updateMethod=DISCRETE
  data: ax input; Thr input; slip input; AdjThr input; y output; threshold input; dbg output
function [y,dbg] = fcn(ax, Thr,slip,AdjThr,threshold)

if Thr > 0 && ax >0 && slip > threshold 
    if AdjThr > 0
        AdjThr = 0;
    end
    y = AdjThr+Thr;
    dbg = 1;   
else
    
    y = Thr;
    %For later, try without this line
    dbg = 0;
end

== matlab function SD2231_Lab1_2022/CarMaker/Your ABS Controller/Activation Logic Br RR/Subsystem/PID1/MATLAB Function ==
  data: threshold_br_r input; slip input; Brk input; res output
function res = fcn(threshold_br_r, slip, Brk)
if Brk >0 && slip > threshold_br_r
    res = 1;
else
    res = 0;
end
end

== matlab function SD2231_Lab1_2022/CarMaker/Your ABS Controller/Activation Logic Br FR/Subsystem1/PID1/MATLAB Function1 ==
  data: threshold_br_r input; slip input; Brk input; res output
function res = fcn(threshold_br_r, slip, Brk)
if Brk >0 && slip > threshold_br_r
    res = 1;
else
    res = 0;
end
end

== matlab function SD2231_Lab1_2022/CarMaker/Road friction/MATLAB Function ==
  data: vx input; mu output; ax input
function mu = fcn(vx, ax)
    if vx > 10 && ax > 0 && vx<20
        mu = 0.7;
    elseif vx < 10 && ax <-0.3 
        mu = 0.3;
    else
        mu = 1;
    end

== matlab function SD2231_Lab1_2022/CarMaker/Your Traction Controller/Activation Logic Tr RR/Controller/MATLAB Function ==
  data: Brk input; res output
function res = fcn(Brk)
if Brk >0
    res = 1;
else
    res = 0;
end
end

== matlab function SD2231_Lab1_2022/CarMaker/Your Traction Controller/Activation Logic Tr RR/MATLAB Function ==
  data: ax input; Thr input; slip input; AdjThr input; y output; threshold input
    function y = fcn(ax, Thr,slip,AdjThr, threshold)
if Thr > 0 && ax >0 && slip > threshold 
    if AdjThr >0
        AdjThr = 0;
    end
    
    y = AdjThr+Thr;
else 
    y = Thr; %For later, try without this line
end

== matlab function SD2231_Lab1_2022/CarMaker/Your ABS Controller/Activation Logic Br FL/MATLAB Function ==
  data: vx input; ax input; Brk input; slip input; AdjBrk input; y output; threshold input; vx_threshold input
function y = fcn(vx, ax, Brk,slip,AdjBrk, threshold,vx_threshold)
if Brk > 0 && ax <0 && slip > threshold && vx > vx_threshold
    if AdjBrk > 0
        AdjBrk = 0;
    end
    y = AdjBrk+Brk;
else 
    y = Brk; %For later, try without this line
end

== matlab function SD2231_Lab1_2022/CarMaker/Your ABS Controller/Activation Logic Br FL/Subsystem/PID1/MATLAB Function ==
  data: threshold_br_r input; slip input; Brk input; res output
function res = fcn(threshold_br_r, slip, Brk)
if Brk >0 && slip > threshold_br_r
    res = 1;
else
    res = 0;
end
end

== matlab function SD2231_Lab1_2022/CarMaker/Your Traction Controller/Activation Logic Tr RL/Subsystem/PID/MATLAB Function1 ==
  data: Thr input; res output; threshold input; slip input
function res = fcn(Thr,threshold,slip)
if Thr >0 && slip > threshold
    res = 1;
else
    res = 0;
end
end

== matlab function SD2231_Lab1_2022/CarMaker/Your ABS Controller/Activation Logic Br RR old 2/MATLAB Function ==
  data: vx input; ax input; Brk input; slip input; AdjBrk input; y output; threshold input; vx_threshold input
function y = fcn(vx, ax, Brk,slip,AdjBrk, threshold,vx_threshold)
if Brk > 0 && ax <0 && slip > threshold && vx > vx_threshold
        if AdjBrk > 0
            AdjBrk = 0;
        end
    y = AdjBrk+Brk;
else 
    y = Brk; %For later, try without this line
end
